simulink model "BACKUPCmdVelPub"  (R2022a)
settings: Solver=FixedStepAuto  StartTime=0  StopTime=inf  FixedStep=0.1  RelTol=1e-3
values from neighbouring files (symbols this model uses):
  tN = (tO(1):dt:tO(end)).' - tO(1)    [A2_Publishing.m]    (also in A3_VelocitySmoothing.m; A4_VelocitySmoothing.m)
  VAN = VA(1:3:length(VA))    [A2_Publishing.m]    (also in A3_VelocitySmoothing.m = CVAtris(1:3:length(CVAtris)); A4_VelocitySmoothing.m = CVAtris(1:3:length(CVAtris)))
  VLN = VL(1:3:length(VL))    [A2_Publishing.m]    (also in A3_VelocitySmoothing.m = CVLtris(1:3:length(CVLtris)); A4_VelocitySmoothing.m = CVLtris(1:3:length(CVLtris)))
undefined symbols (not defined in the file or in its folder): Angular, Linear
libraries: robotlib x10
settings Model: Creator=jacopo  LastModifiedBy=jacopo
settings OptimizationCC: EnhancedBackFolding=on  PassReuseOutputArgsAs=Individual arguments  ZeroExternalMemoryAtStartup=off  ZeroInternalMemoryAtStartup=off  MaxStackSize=64  OptimizeBlockOrder=speed  DifferentSizesBufferReuse=on  OptimizationCustomize=off  EfficientTunableParamExpr=on
settings DebuggingCC: ParameterTunabilityLossMsg=error
settings HardwareCC: ProdBitPerPointer=32  ProdBitPerSizeT=32  ProdBitPerPtrDiffT=32  ProdLargestAtomicFloat=None  ProdIntDivRoundTo=Undefined  ProdEndianess=Unspecified  ProdWordSize=32  ProdHWDeviceType=Generic->Unspecified (assume 32-bit Generic)
settings SFSimCC: MATLABDynamicMemAlloc=off
settings RTWCC: SystemTargetFile=ert.tlc  HardwareBoard=Robot Operating System (ROS)  TLCOptions="-aInlineSetEventsForThisBaseRateFcn=TLC_FALSE -aSuppressMultiTaskScheduler=TLC_FALSE  -aRateBasedStepFcn=0"  TemplateMakefile=ert_default_tmf  Toolchain=Catkin  TargetLang=C++
settings CodeAppCC: ForceParamTrailComments=on  IgnoreCustomStorageClasses=off  OperatorAnnotations=on  SimulinkDataObjDesc=on  SFDataObjDesc=on  InsertBlockDesc=on

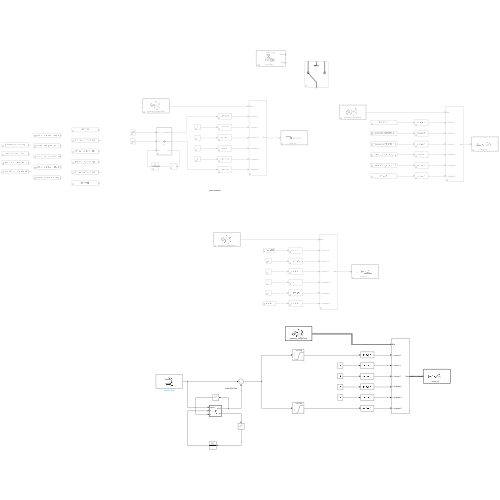
[thumbnail: Simulink's stored preview of the top-level diagram]
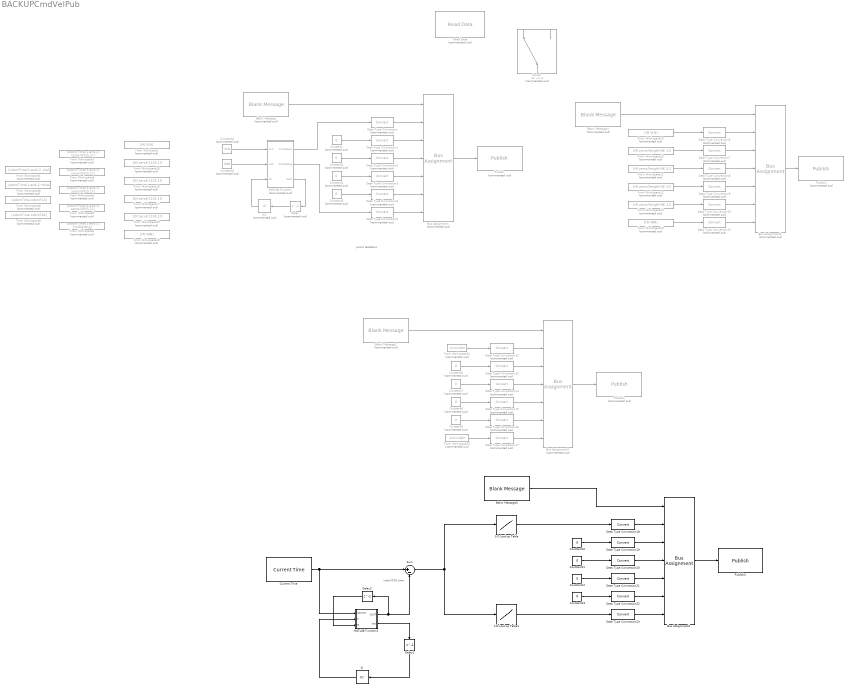
== system BACKUPCmdVelPub ==
  note: primo tentativo
  note: initial ROS time
  1-D Lookup Table : Lookup_n-D  NumberOfTableDimensions=1  BreakpointsForDimension1=tN  Table=VLN  InternalRulePriority=Speed  RndMeth=Simplest
  1-D Lookup Table1 : Lookup_n-D  NumberOfTableDimensions=1  BreakpointsForDimension1=tN  Table=VAN  InternalRulePriority=Speed  RndMeth=Simplest
  Blank Message : robotlib/Blank Message  Commented=on  messageClass=Message  entityType=geometry_msgs/Twist  messageType=geometry_msgs/Twist  SampleTime=inf  legacyBusStruct=off
  Blank Message1 : robotlib/Blank Message  Commented=on  messageClass=Message  entityType=geometry_msgs/Twist  messageType=geometry_msgs/Twist  SampleTime=inf  legacyBusStruct=off
  Blank Message2 : robotlib/Blank Message  Commented=on  messageClass=Message  entityType=geometry_msgs/Twist  messageType=geometry_msgs/Twist  SampleTime=inf  legacyBusStruct=off
  Blank Message3 : robotlib/Blank Message  messageClass=Message  entityType=geometry_msgs/Twist  messageType=geometry_msgs/Twist  SampleTime=inf  legacyBusStruct=off
  Bus Assignment : BusAssignment  Commented=on  AssignedSignals=Linear.X,Linear.Y,Linear.Z,Angular.X,Angular.Y,Angular.Z
  Bus Assignment1 : BusAssignment  Commented=on  AssignedSignals=Linear.X,Linear.Y,Linear.Z,Angular.X,Angular.Y,Angular.Z
  Bus Assignment2 : BusAssignment  Commented=on  AssignedSignals=Linear.X,Linear.Y,Linear.Z,Angular.X,Angular.Y,Angular.Z
  Bus Assignment3 : BusAssignment  AssignedSignals=Linear.X,Linear.Y,Linear.Z,Angular.X,Angular.Y,Angular.Z
  Constant{,1..3,6..9} (8 alike) : Constant  Commented=on  Value=0
  Constant{10..13} (4 alike) : Constant  Value=0
  Constant4 : Constant  Commented=on  Value=VLN
  Constant5 : Constant  Commented=on  Value=VAN
  Current Time : robotlib/Current Time  OutputFormat=double  SampleTime=-1  ModelName=CmdVelPub
      settings: SourceProductBaseCode=RR
  Data Type Conversion{,1..17} (18 alike) : DataTypeConversion  Commented=on  SaturateOnIntegerOverflow=off  RndMeth=Floor
  Data Type Conversion{18..23} (6 alike) : DataTypeConversion  SaturateOnIntegerOverflow=off  RndMeth=Floor
  Delay : Delay  Commented=on  DelayLength=1
  Delay1 : Delay  DelayLength=1
  Delay2 : Delay  DelayLength=1
  From Workspace : FromWorkspace  Commented=on  VariableName=[tN VLN]
  From Workspace1 : FromWorkspace  Commented=on  VariableName=[odomTime(1:end-1) yVel]
  From Workspace10 : FromWorkspace  Commented=on  VariableName=[tN VLN]
  From Workspace{11..12,14..15} (4 alike) : FromWorkspace  Commented=on  VariableName=[tN zeros(length(tN),1)]
  From Workspace13 : FromWorkspace  Commented=on  VariableName=[tN VAN]
  From Workspace{16..19} (4 alike) : FromWorkspace  Commented=on  VariableName=[tN zeros(1105,1)]
  From Workspace{2..3,5,7} (4 alike) : FromWorkspace  Commented=on  VariableName=[odomTime(1:end-1) zeros(3315,1)]
  From Workspace20 : FromWorkspace  Commented=on  VariableName=[tN VAN]
  From Workspace21 : FromWorkspace  Commented=on  VariableName=siminVLN
  From Workspace22 : FromWorkspace  Commented=on  VariableName=siminVAN
  From Workspace4 : FromWorkspace  Commented=on  VariableName=[odomTime(1:end-1) CmdVelAng]
  From Workspace6 : FromWorkspace  Commented=on  VariableName=[odomTime(1:end-1) thVel]
  From Workspace8 : FromWorkspace  Commented=on  VariableName=[odomTime odomTLX]
  From Workspace9 : FromWorkspace  Commented=on  VariableName=[odomTime odomTAX]
  IC : InitialCondition
  IC1 : InitialCondition  Commented=on
  MATLAB Function : MATLAB Function  Commented=on  TreatAsAtomicUnit=on
  MATLAB Function1 : MATLAB Function  TreatAsAtomicUnit=on
  Publish : robotlib/Publish  Commented=on  topicSource=Select from ROS network  topic=/cmd_vel  messageType=geometry_msgs/Twist  legacyBusStruct=off  messageQueueLength=1
  Publish1 : robotlib/Publish  Commented=on  topicSource=Select from ROS network  topic=/cmd_vel  messageType=geometry_msgs/Twist  legacyBusStruct=off  messageQueueLength=1
  Publish2 : robotlib/Publish  Commented=on  topicSource=Select from ROS network  topic=/cmd_vel  messageType=geometry_msgs/Twist  legacyBusStruct=off  messageQueueLength=1
  Publish3 : robotlib/Publish  topicSource=Select from ROS network  topic=/cmd_vel  messageType=geometry_msgs/Twist  legacyBusStruct=off  messageQueueLength=1
  Read Data : robotlib/Read Data  Commented=on  topic=/my_topic  sampleTime=-1  logfileType=rosbag  modelName=CmdVelPub
      settings: SourceProductBaseCode=RR
  Sum : Sum  Inputs=|+-
  Switch : Switch  Commented=on  Criteria=u2 ~= 0  SaturateOnIntegerOverflow=off  InputSameDT=off
  wires:
  Blank Message/1 -> Bus Assignment/1
  Bus Assignment/1 -> Publish/1
  MATLAB Function/1(CmdVelLon) -> Data Type Conversion/1
  Constant/1 -> Data Type Conversion1/1
  Constant1/1 -> Data Type Conversion2/1
  Constant3/1 -> Data Type Conversion4/1
  Data Type Conversion/1 -> Bus Assignment/2
  Data Type Conversion1/1 -> Bus Assignment/3
  Data Type Conversion2/1 -> Bus Assignment/4
  Data Type Conversion3/1 -> Bus Assignment/5
  Data Type Conversion4/1 -> Bus Assignment/6
  Data Type Conversion5/1 -> Bus Assignment/7
  Constant2/1 -> Data Type Conversion3/1
  MATLAB Function/2(CmdVelAng) -> Data Type Conversion5/1
  From Workspace11/1 -> Data Type Conversion8/1
  Data Type Conversion9/1 -> Bus Assignment1/5
  Data Type Conversion10/1 -> Bus Assignment1/6
  From Workspace10/1 -> Data Type Conversion6/1
  From Workspace13/1 -> Data Type Conversion11/1
  Blank Message1/1 -> Bus Assignment1/1
  Data Type Conversion6/1 -> Bus Assignment1/2
  Bus Assignment1/1 -> Publish1/1
  From Workspace12/1 -> Data Type Conversion9/1
  From Workspace15/1 -> Data Type Conversion7/1
  Data Type Conversion8/1 -> Bus Assignment1/4
  Data Type Conversion11/1 -> Bus Assignment1/7
  Data Type Conversion7/1 -> Bus Assignment1/3
  From Workspace14/1 -> Data Type Conversion10/1
  MATLAB Function/3(IOUT) -> Delay/1
  Delay/1 -> IC1/1
  IC1/1 -> MATLAB Function/3(IIN)
  Constant4/1 -> MATLAB Function/1(VLN)
  Constant5/1 -> MATLAB Function/2(VAN)
  Sum/1 -> 1-D Lookup Table/1, 1-D Lookup Table1/1
  Current Time/1 -> Sum/1, MATLAB Function1/1(rostime)
  Bus Assignment2/1 -> Publish2/1
  Data Type Conversion12/1 -> Bus Assignment2/2
  Data Type Conversion15/1 -> Bus Assignment2/5
  Data Type Conversion17/1 -> Bus Assignment2/7
  Data Type Conversion14/1 -> Bus Assignment2/4
  Data Type Conversion13/1 -> Bus Assignment2/3
  Data Type Conversion16/1 -> Bus Assignment2/6
  Constant9/1 -> Data Type Conversion16/1
  Constant7/1 -> Data Type Conversion14/1
  Constant6/1 -> Data Type Conversion13/1
  Constant8/1 -> Data Type Conversion15/1
  Blank Message2/1 -> Bus Assignment2/1
  From Workspace21/1 -> Data Type Conversion12/1
  From Workspace22/1 -> Data Type Conversion17/1
  Data Type Conversion18/1 -> Bus Assignment3/2
  Bus Assignment3/1 -> Publish3/1
  Constant10/1 -> Data Type Conversion19/1
  Blank Message3/1 -> Bus Assignment3/1
  Constant12/1 -> Data Type Conversion21/1
  Constant13/1 -> Data Type Conversion22/1
  Data Type Conversion19/1 -> Bus Assignment3/3
  Data Type Conversion22/1 -> Bus Assignment3/6
  Data Type Conversion20/1 -> Bus Assignment3/4
  Data Type Conversion23/1 -> Bus Assignment3/7
  Data Type Conversion21/1 -> Bus Assignment3/5
  Constant11/1 -> Data Type Conversion20/1
  1-D Lookup Table1/1 -> Data Type Conversion23/1
  1-D Lookup Table/1 -> Data Type Conversion18/1
  MATLAB Function1/2(out) -> Delay1/1
  Delay1/1 -> IC/1
  IC/1 -> MATLAB Function1/2(in)
  MATLAB Function1/1(tOUT) -> Delay2/1, Sum/2
  Delay2/1 -> MATLAB Function1/3(t0)

== matlab function BACKUPCmdVelPub/MATLAB Function1 ==
  data: rostime input; tOUT output; in input; out output; t0 input
function [tOUT, out] = fcn(rostime, in, t0)


if in == 1
    tOUT = rostime;
    out = 0;
else
    tOUT = t0;
    out = 0;
end

== matlab function BACKUPCmdVelPub/MATLAB Function ==
  data: VLN input; CmdVelLon output; VAN input; IIN input; CmdVelAng output; IOUT output
function [CmdVelLon, CmdVelAng, IOUT]    = fcn(VLN, VAN, IIN)

CmdVelLon = VLN(IIN);
CmdVelAng = VAN(IIN);
IOUT = IIN + 1;
